simulink model "BuckConverter"  (R2019a)
settings: Solver=VariableStepAuto  StartTime=0.0  StopTime=0.5  RelTol=1e-3
libraries: powerlib x11, powerlib_meascontrol x1
settings Model: Creator=aliaq  LastModifiedBy=aliaq
settings SolverCC: ZeroCrossAlgorithm=Adaptive

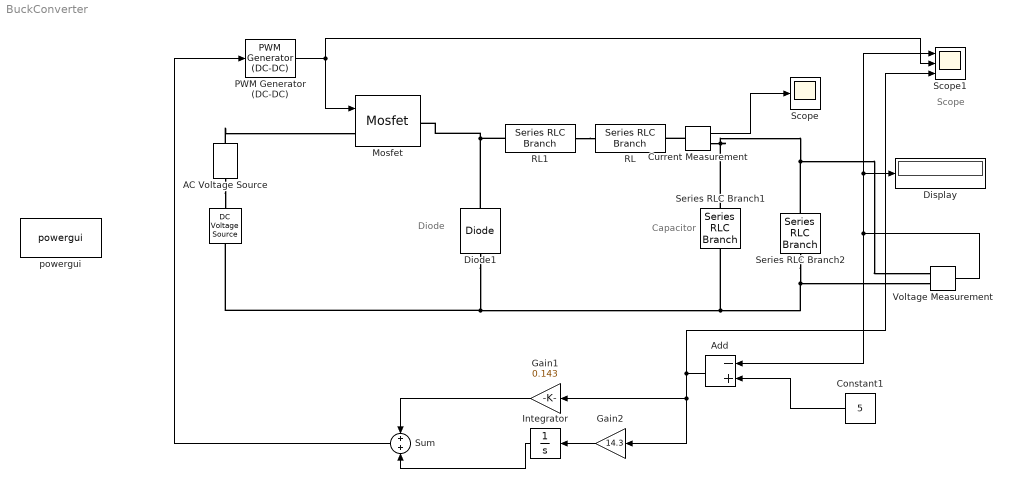
== system BuckConverter ==
  note: Scope
  note: Diode
  note: Capacitor
  " " : powerlib/Electrical Sources/DC Voltage Source  Amplitude=28  Measurements=None
      settings: SourceProductName=Simscape Electrical
  AC Voltage Source : powerlib/Electrical Sources/AC Voltage Source  Amplitude=4  Phase=0  Frequency=5  SampleTime=0  Measurements=None  BusType=swing  Pref=10e3  Qref=0  Qmin=-inf  Qmax=+inf
      settings: SourceProductName=Simscape Electrical
  Add : Sum  Inputs=-+
  Constant1 : Constant  Value=5
  Current Measurement : powerlib/Measurements/Current Measurement  PhasorSimulation=off  OutputType=Complex  PSBequivalent=0
      settings: SourceProductName=Simscape Electrical
  Diode1 : powerlib/Power Electronics/Diode  Ron=0.01  Lon=0  Vf=0  IC=0  UseSnubber=off  Rs=inf  Cs=inf  Measurements=off
      settings: SourceProductName=Simscape Electrical
  Display : Display
  Gain1 : Gain  Gain=0.143
  Gain2 : Gain  Gain=14.3
  Integrator : Integrator
  Mosfet : powerlib/Power Electronics/Mosfet  Ron=1e-3  Lon=0  Rd=1e-3  Vfd=0  IC=0  Rs=inf  Cs=inf  Measurements=off
      settings: SourceProductName=Simscape Electrical
  PWM Generator (DC-DC) : powerlib_meascontrol/Pulse & Signal Generators/PWM Generator (DC-DC)  Fsw=10e3  Ts=0
      settings: SourceProductName=Simscape Electrical
  RL : powerlib/Elements/Series RLC Branch  LConnTagsString=__new0  RConnTagsString=__new0  BranchType=R  Resistance=0.1  Inductance=3e-3  SetiL0=off  InitialCurrent=0  Capacitance=1e-6  Setx0=off  InitialVoltage=0  Measurements=None
      settings: SourceProductName=Simscape Electrical
  RL1 : powerlib/Elements/Series RLC Branch  LConnTagsString=__new0  RConnTagsString=__new0  BranchType=L  Resistance=0.1  Inductance=3e-3  SetiL0=off  InitialCurrent=0  Capacitance=1e-6  Setx0=off  InitialVoltage=0  Measurements=None
      settings: SourceProductName=Simscape Electrical
  Scope : Scope
  Scope1 : Scope  NumInputPorts=3
  Series RLC Branch1 : powerlib/Elements/Series RLC Branch  LConnTagsString=__new0  RConnTagsString=__new0  BranchType=C  Resistance=1e-4  Inductance=200e-6  SetiL0=off  InitialCurrent=0  Capacitance=22e-6  Setx0=off  InitialVoltage=150  Measurements=None
      settings: SourceProductName=Simscape Electrical
  Series RLC Branch2 : powerlib/Elements/Series RLC Branch  LConnTagsString=__new0  RConnTagsString=__new0  BranchType=R  Resistance=5  Inductance=200e-6  SetiL0=off  InitialCurrent=0  Capacitance=30e-6  Setx0=off  InitialVoltage=150  Measurements=None
      settings: SourceProductName=Simscape Electrical
  Sum : Sum
  Voltage Measurement : powerlib/Measurements/Voltage Measurement  PhasorSimulation=off  OutputType=Complex  PSBequivalent=0
      settings: SourceProductName=Simscape Electrical
  powergui : powerlib/powergui  Priority=1  SimulationMode=Continuous  SampleTime=50e-6  frequency=60  Iterations=50  frequencyindice=0  Pbase=100e6  ErrMax=1e-4  UnitsV=kV  UnitsW=MW  buscounter=0  FunctionMessages=off  echomessages=off  EnableUseOfTLC=off  CurrentSourceSwitches=off  DisableSnubberDevices=off  DisableRonSwitches=off  DisableVfSwitches=off  DisplayEquations=off  AutomaticDiscreteSolvers=off  SolverType=Tustin/Backward Euler (TBE)  Interpol=off  ExternalGateDelay=off  methode=off  Ts=100  x0status=blocks  SPID=on  SwTol=0  HookPort=off  NonlinearTolerance=0  nMaxIteration=15  ContinueOnMaxIteration=off  RestoreLinks=warning  ResistiveCurrentMeasurement=off  Frange=[0:2:500]  Ylog=off  Xlog=on  ShowGrid=off  save=off  variable=ZData  structure=0  ZoomFFT=off  StartTime=0.0  cycles=1  DisplayStyle=1  fundamental=60  FreqAxis=off  MaxFrequency=1000  frequencyindicesteady=1  RmsSteady=1  display=off
      settings: SourceProductName=Simscape Electrical
  wires:
  PWM Generator (DC-DC)/1 -> Mosfet/1, Scope1/2
  Constant1/1 -> Add/2
  Voltage Measurement/1 -> Display/1, Scope1/1, Add/1
  Current Measurement/1 -> Scope/1
  Add/1 -> Scope1/3, Gain2/1, Gain1/1
  Gain1/1 -> Sum/1
  Integrator/1 -> Sum/2
  Gain2/1 -> Integrator/1
  Sum/1 -> PWM Generator (DC-DC)/1
  connections:
  Diode1/RConn1 -- RL1/LConn1 -- Mosfet/RConn1
  Series RLC Branch1/LConn1 -- Current Measurement/RConn1 -- Series RLC Branch2/LConn1 -- Voltage Measurement/LConn1
  Diode1/LConn1 -- " "/LConn1 -- Series RLC Branch1/RConn1 -- Series RLC Branch2/RConn1 -- Voltage Measurement/LConn2
  Current Measurement/LConn1 -- RL/RConn1
  AC Voltage Source/LConn1 -- " "/RConn1
  AC Voltage Source/RConn1 -- Mosfet/LConn1
  RL1/RConn1 -- RL/LConn1
